simulink model "test_sys"  (R2022b)
settings: Solver=FixedStepDiscrete  StartTime=0.0  StopTime=T_final  FixedStep=T_sample  RelTol=1e-3
values from neighbouring files (symbols this model uses):
  A = [0.995 0.0998 ... (first row only)    [Run_model.m]
  B = [0.1; 0.1]    [Run_model.m]
  C = [0.571052826934  0.00320705121121; 0.105905694945  0.429437411805; 0.715489520193  0.338935563141; 0.31761476712  0.78571602684; 0.688586017165  0.771120435927; 0.876557849311  0.658449257994]    [C.mat]    (also in Run_model.m = load('C.mat'))
  D = zeros(n_meas,n_int)    [Run_model.m]
  x0 = 7*ones(n_states,1)    [Run_model.m]
settings Model: Creator=Abelb  LastModifiedBy=Abelb
settings DebuggingCC: UnconnectedInputMsg=warning  UnconnectedOutputMsg=warning  UnconnectedLineMsg=warning
settings ModelReferenceCC: EnableRefExpFcnMdlSchedulingChecks=on
settings RTWCC: DLArmComputeVersion=19.05

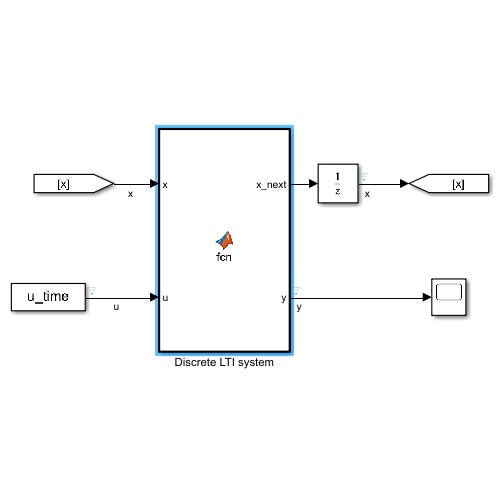
[thumbnail: Simulink's stored preview of the top-level diagram]
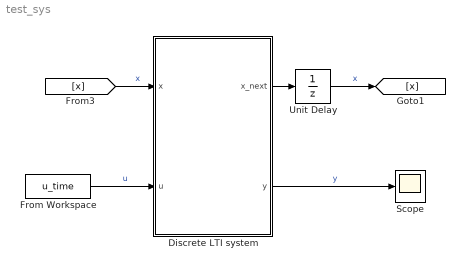
== system test_sys ==
  Discrete LTI system : MATLAB Function  TreatAsAtomicUnit=on
  From Workspace : FromWorkspace  VariableName=u_time
  Scope : Scope
  Unit Delay : UnitDelay  InitialCondition=x0  SampleTime=-1  HasFrameUpgradeWarning=on
  wires:
  Discrete LTI system/1(x_next) -> Unit Delay/1
  From Workspace/1 -> Discrete LTI system/2(u)  "u"
  Unit Delay/1 -> [x]  "x"
  [x] -> Discrete LTI system/1(x)  "x"
  Discrete LTI system/2(y) -> Scope/1  "y"

== matlab function test_sys/Discrete LTI system ==
  data: x input; x_next output; u input; y output; A parameter; C parameter; B parameter; D parameter
function [x_next,y] = fcn(x,u,A,C,B,D)
% Discrete state-space model for system

x_next = A*x + B*u;

y = C*x + D*u;
